simulink model "SP_linear_LQG_controller"  (R2016b)
settings: Solver=ode8  StartTime=0.0  StopTime=10  FixedStep=0.01  RelTol=1e-3
values from neighbouring files (symbols this model uses):
  A2_TM = [-0.593423370112  9.03046955965; 0.145010309281  -0.463845505604]    [SP_linsys_TM.mat]
  Aol = [0 C;zeros(2,1) A]    [SP_LQG_controller_design.m]
  B2_TM = [-0.0230170398372 -0.156555660268]    [SP_linsys_TM.mat]
  Bol = [0;B]    [SP_LQG_controller_design.m]
  C2_TM = [1.01502313109 0]    [SP_linsys_TM.mat]
  Col = [Ke_sp Kx_sp]    [SP_LQG_controller_design.m]
  Ke_sp = K_bar(:,1)    [SP_LQG_controller_design.m]    (also in controller_parameter.mat = -14.1421356237)
  Kx_sp = K_bar(:,2:end)    [SP_LQG_controller_design.m]    (also in controller_parameter.mat = [-9.4028503548 -29.2130812278])
libraries: simulink x1
settings Model: Creator=whn  LastModifiedBy=whn

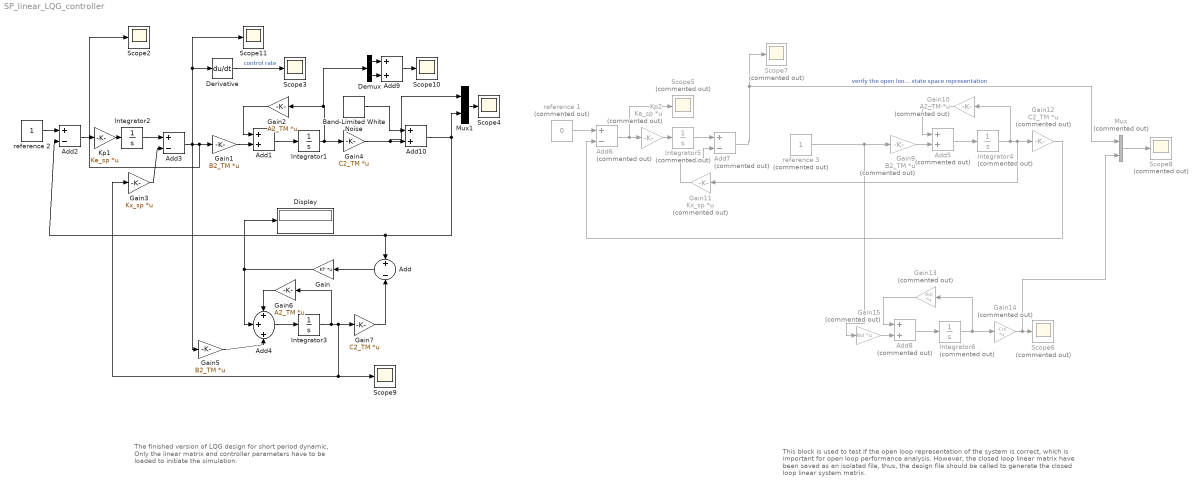
== system SP_linear_LQG_controller ==
  note: This block is used to test if the open loop representation of the system is correct,
      | which is important for open loop performance analysis. However, the closed loop
      | linear matrix have been saved as an isolated file, thus, the design file should be called
      | to generate the closed loop linear system matrix.
  note: The finished version of LQG design for short period dynamic,
      | Only the linear matrix and controller parameters have to be
      | loaded to initiate the simulation.
  Add : Sum  Inputs=+-
  Add1 : Sum
  Add10 : Sum
  Add2 : Sum  Inputs=+-
  Add3 : Sum  Inputs=+-
  Add4 : Sum  Inputs=+++
  Add5 : Sum  Commented=on
  Add6 : Sum  Commented=on  Inputs=+-
  Add7 : Sum  Commented=on  Inputs=+-
  Add8 : Sum  Commented=on
  Add9 : Sum
  Band-Limited White Noise : simulink/Sources/Band-Limited White Noise  Cov=1e-5  Ts=0.01  seed=[23341]
  Demux : Demux  Outputs=2
  Derivative : Derivative
  Display : Display
  Gain : Gain  Gain=Kf'  Multiplication=Matrix(K*u)
  Gain1 : Gain  Gain=B2_TM  Multiplication=Matrix(K*u)
  Gain10 : Gain  Commented=on  Gain=A2_TM  Multiplication=Matrix(K*u)
  Gain11 : Gain  Commented=on  Gain=Kx_sp  Multiplication=Matrix(K*u)
  Gain12 : Gain  Commented=on  Gain=C2_TM  Multiplication=Matrix(K*u)
  Gain13 : Gain  Commented=on  Gain=Aol  Multiplication=Matrix(K*u)
  Gain14 : Gain  Commented=on  Gain=-Col  Multiplication=Matrix(K*u)
  Gain15 : Gain  Commented=on  Gain=Bol  Multiplication=Matrix(K*u)
  Gain2 : Gain  Gain=A2_TM  Multiplication=Matrix(K*u)
  Gain3 : Gain  Gain=Kx_sp  Multiplication=Matrix(K*u)
  Gain4 : Gain  Gain=C2_TM  Multiplication=Matrix(K*u)
  Gain5 : Gain  Gain=B2_TM  Multiplication=Matrix(K*u)
  Gain6 : Gain  Gain=A2_TM  Multiplication=Matrix(K*u)
  Gain7 : Gain  Gain=C2_TM  Multiplication=Matrix(K*u)
  Gain9 : Gain  Commented=on  Gain=B2_TM  Multiplication=Matrix(K*u)
  Integrator1 : Integrator
  Integrator2 : Integrator
  Integrator3 : Integrator
  Integrator4 : Integrator  Commented=on
  Integrator5 : Integrator  Commented=on
  Integrator6 : Integrator  Commented=on
  Kp1 : Gain  Gain=Ke_sp  Multiplication=Matrix(K*u)
  Kp2 : Gain  Commented=on  Gain=Ke_sp  Multiplication=Matrix(K*u)
  Mux : Mux  Commented=on  Inputs=2
  Mux1 : Mux  Inputs=2
  Scope{2..4,9..11} (6 alike) : Scope
  Scope{5..8} (4 alike) : Scope  Commented=on
  reference 1 : Constant  Commented=on  Value=0
  reference 2 : Constant
  reference 3 : Constant  Commented=on
  wires:
  Gain1/1 -> Add1/2
  Add1/1 -> Integrator1/1
  Gain2/1 -> Add1/1
  Gain3/1 -> Add3/2
  Add2/1 -> Kp1/1
  Kp1/1 -> Integrator2/1
  reference 2/1 -> Add2/1
  Integrator2/1 -> Add3/1
  Add3/1 -> Gain5/1, Scope2/1, Gain1/1, Scope11/1, Derivative/1
  Gain5/1 -> Add4/3
  Add4/1 -> Integrator3/1
  Gain6/1 -> Add4/1
  Derivative/1 -> Scope3/1  "control rate"
  Gain7/1 -> Add/2
  Add/1 -> Gain/1
  Gain/1 -> Display/1, Add4/2
  Gain9/1 -> Add5/2
  Add5/1 -> Integrator4/1
  Gain10/1 -> Add5/1
  Gain11/1 -> Add7/2
  Integrator4/1 -> Gain10/1, Gain12/1, Gain11/1
  Gain12/1 -> Add6/2
  Add6/1 -> Kp2/1, Scope5/1
  Kp2/1 -> Integrator5/1
  reference 1/1 -> Add6/1
  Integrator5/1 -> Add7/1
  Add7/1 -> Mux/1, Scope7/1  "verify the open loop state space representation"
  reference 3/1 -> Gain9/1, Gain15/1
  Gain15/1 -> Add8/2
  Add8/1 -> Integrator6/1
  Gain13/1 -> Add8/1
  Integrator6/1 -> Gain13/1, Gain14/1
  Gain14/1 -> Mux/2, Scope6/1
  Mux/1 -> Scope8/1
  Integrator1/1 -> Gain4/1, Demux/1, Gain2/1
  Demux/2 -> Add9/2
  Demux/1 -> Add9/1
  Add9/1 -> Scope10/1
  Band-Limited White Noise/1 -> Add10/1
  Integrator3/1 -> Gain6/1, Scope9/1, Gain3/1, Gain7/1
  Add10/1 -> Add2/2, Add/1, Mux1/2
  Mux1/1 -> Scope4/1
  Gain4/1 -> Mux1/1, Add10/2
